simulink model "Bait_Ambrosino_place"  (R2025b)
settings: Solver=VariableStepAuto  StartTime=0.0  StopTime=10.0  RelTol=1e-3
undefined symbols (not defined in the file): A, B, C, Comp, K_place, nu, nx, x0, xref
settings Model: Creator=Miche  LastModifiedBy=Miche

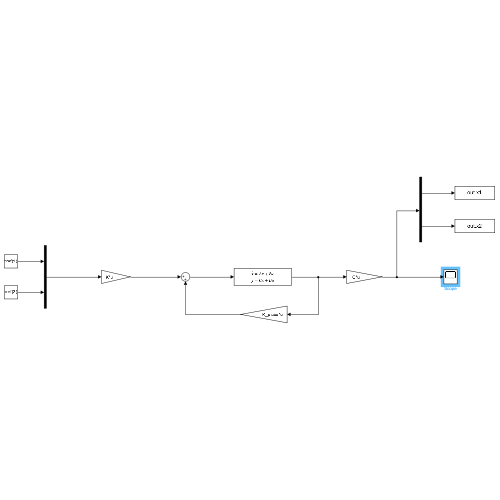
[thumbnail: Simulink's stored preview of the top-level diagram]
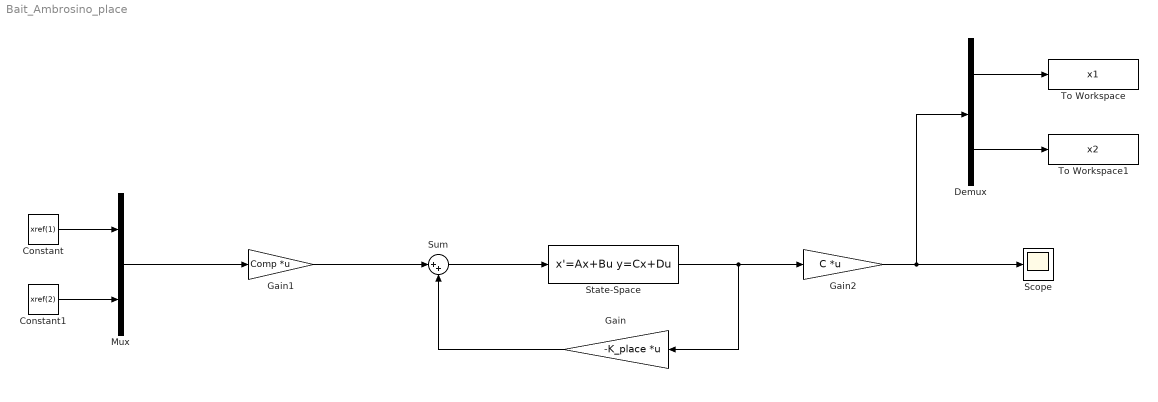
== system Bait_Ambrosino_place ==
  Constant : Constant  Value=xref(1)
  Constant1 : Constant  Value=xref(2)
  Demux : Demux  Outputs=2
  Gain : Gain  Gain=-K_place  Multiplication=Matrix(K*u)
  Gain1 : Gain  Gain=Comp  Multiplication=Matrix(K*u)
  Gain2 : Gain  Gain=C  Multiplication=Matrix(K*u)
  Mux : Mux  Inputs=2
  Scope : Scope
      settings: ActiveDisplayYMinimum=-0.012499999999999969  ActiveDisplayYMaximum=1.1125
  State-Space : StateSpace  A=A  B=B  C=eye(nx)  D=zeros(nx,nu)  InitialCondition=x0
  Sum : Sum  Inputs=|++
  To Workspace : ToWorkspace  VariableName=x1  SaveFormat=Timeseries  SampleTime=-1
  To Workspace1 : ToWorkspace  VariableName=x2  SaveFormat=Timeseries  SampleTime=-1
  wires:
  Sum/1 -> State-Space/1
  Gain/1 -> Sum/2
  Gain1/1 -> Sum/1
  Mux/1 -> Gain1/1
  Constant/1 -> Mux/1
  Constant1/1 -> Mux/2
  State-Space/1 -> Gain/1, Gain2/1
  Gain2/1 -> Demux/1, Scope/1
  Demux/1 -> To Workspace/1
  Demux/2 -> To Workspace1/1
